simulink model "app_Main100msMgr"  (R2016b)
settings: Solver=FixedStepDiscrete  StartTime=0.0  StopTime=10.0  FixedStep=0.001  RelTol=1e-3  EnableMultiTasking=on
PreLoadFcn:
  | try
  |    tapas_types('load');
  | catch
  |   disp('TAPAS WARNING: Tapas Types could not be loaded ...');
  | end
  | 
  | try
  |   app_types('load');
  | catch
  |   currdir =pwd;
  |   try
  |     cd('..\app_types\');
  |     app_types('load');
  |     cd(currdir);
  |   catch
  |     try
  |        cd('..\..\app_types\');
  |        app_types('load');
  |        cd(currdir);
  |     catch
  |        cd(currdir);
  |        disp('TAPAS WARNING: Application Types could not be loaded ...');
  |     end
  |   end
  |   try
  |       clear currdir;
  |   catch
  |      %Do nothing
  |   end
  | end
libraries: Lib_ICAT_VCU_Com x76, Lib_ICAT_VCU_IO x12, simulink x2, Lib_ICAT_VCU_Anlg x1
(part 1 of 2)
settings Model: Creator=kmansour  LastModifiedBy=Santosh
settings DataIOCC: LimitDataPoints=on  SaveFormat=Array
settings OptimizationCC: LifeSpan=1
settings DebuggingCC: AllowSymbolicDim=off  SFUnexpectedBacktrackingDiag=warning  SFNoUnconditionalDefaultTransitionDiag=warning  SFExecutionAtInitializationDiag=none
settings HardwareCC: ProdBitPerPointer=32  ProdBitPerSizeT=32  ProdBitPerPtrDiffT=32  ProdLargestAtomicInteger=Long  ProdLargestAtomicFloat=Double  ProdWordSize=32  ProdHWDeviceType=Texas Instruments->TMS570 Cortex-R4
settings ModelReferenceCC: ModelReferenceNumInstancesAllowed=Single  PropagateSignalLabelsOutOfModel=off
settings RTWCC: SystemTargetFile=ert.tlc  GenCodeOnly=on  TemplateMakefile=ert_default_tmf  Description=Embedded Coder  GenerateReport=on  IncludeHyperlinkInReport=on  LaunchReport=on  GenerateTraceInfo=on  GenerateTraceReport=on  GenerateTraceReportSl=on  GenerateTraceReportSf=on  GenerateTraceReportEml=on
settings CodeAppCC: IgnoreCustomStorageClasses=off  MaxIdLength=63
settings ERTTargetCC: GenerateSampleERTMain=on  ERTSrcFileBannerTemplate=tapas_code_template.cgt  ERTHdrFileBannerTemplate=tapas_code_template.cgt  ERTDataSrcFileTemplate=tapas_code_template.cgt  ERTDataHdrFileTemplate=tapas_code_template.cgt  ERTCustomFileTemplate=example_file_process.tlc  ConvertIfToSwitch=off  SuppressUnreachableDefaultCases=off
settings ConfigComp: CovMetricSettings=dw  CovHtmlReporting=on  CovSaveCumulativeToWorkspaceVar=on  CovSaveSingleToWorkspaceVar=on  CovExternalEMLEnable=off

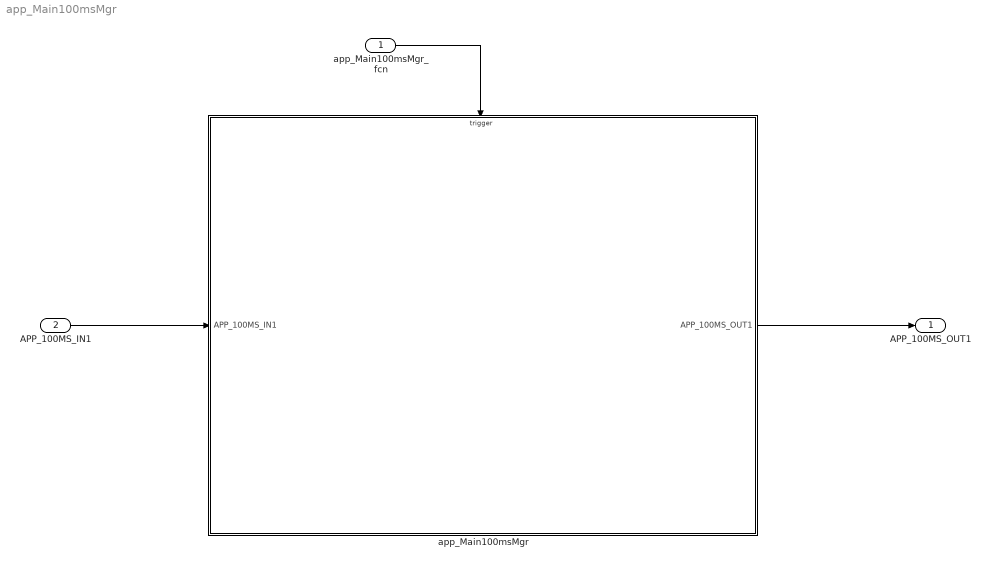
== system app_Main100msMgr ==
  app_Main100msMgr_fcn : Inport  SampleTime=100e-3  OutputFunctionCall=on
  APP_100MS_IN1 : Inport  Port=2
  app_Main100msMgr : Subsystem
  APP_100MS_OUT1 : Outport
  wires:
  app_Main100msMgr_fcn/1 -> app_Main100msMgr/Trigger
  APP_100MS_IN1/1 -> app_Main100msMgr/1(APP_100MS_IN1)
  app_Main100msMgr/1(APP_100MS_OUT1) -> APP_100MS_OUT1/1

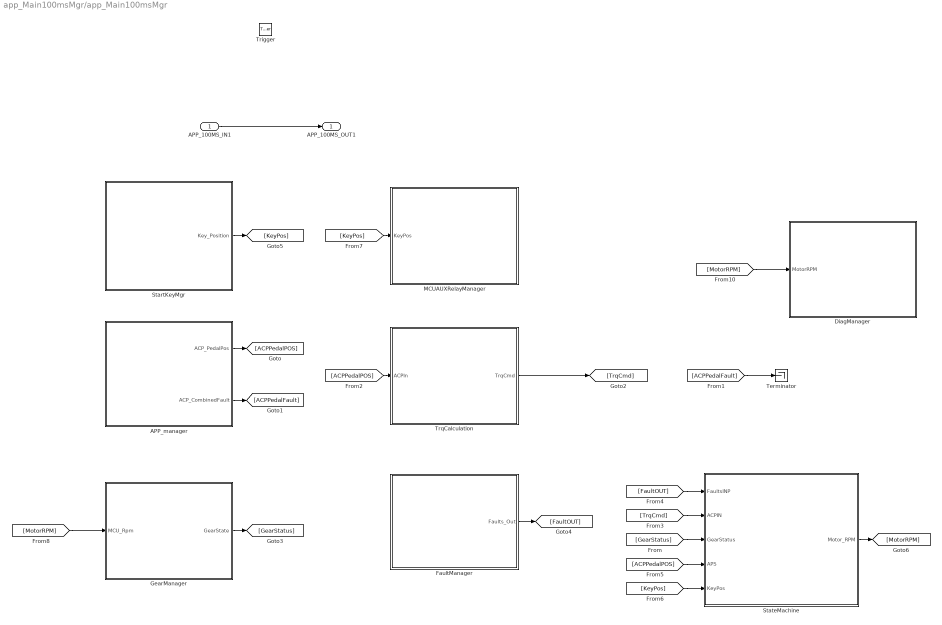
== system app_Main100msMgr/app_Main100msMgr ==
  APP_100MS_IN1 : Inport
  Trigger : TriggerPort  TriggerType=function-call  VariantControl=Variant  SampleTimeType=periodic  SampleTime=-1  PortDimensions=1
  APP_manager : Subsystem
  DiagManager : Subsystem
  FaultManager : Subsystem
  GearManager : Subsystem
  MCUAUXRelayManager : Subsystem
  StartKeyMgr : Subsystem
  StateMachine : Subsystem
  Terminator : Terminator
  TrqCalculation : Subsystem
  APP_100MS_OUT1 : Outport
  wires:
  APP_100MS_IN1/1 -> APP_100MS_OUT1/1
  [ACPPedalPOS] -> StateMachine/4(APS)
  [TrqCmd] -> StateMachine/2(ACPIN)
  [FaultOUT] -> StateMachine/1(FaultsINP)
  [ACPPedalPOS] -> TrqCalculation/1(ACPIn)
  [ACPPedalFault] -> Terminator/1
  GearManager/1(GearState) -> [GearStatus]
  StartKeyMgr/1(Key_Position) -> [KeyPos]
  [KeyPos] -> MCUAUXRelayManager/1(KeyPos)
  [GearStatus] -> StateMachine/3(GearStatus)
  APP_manager/2(ACP_CombinedFault) -> [ACPPedalFault]
  [MotorRPM] -> GearManager/1(MCU_Rpm)
  [MotorRPM] -> DiagManager/1(MotorRPM)
  APP_manager/1(ACP_PedalPos) -> [ACPPedalPOS]
  TrqCalculation/1(TrqCmd) -> [TrqCmd]
  StateMachine/1(Motor_RPM) -> [MotorRPM]
  FaultManager/1(Faults_Out) -> [FaultOUT]
  [KeyPos] -> StateMachine/5(KeyPos)

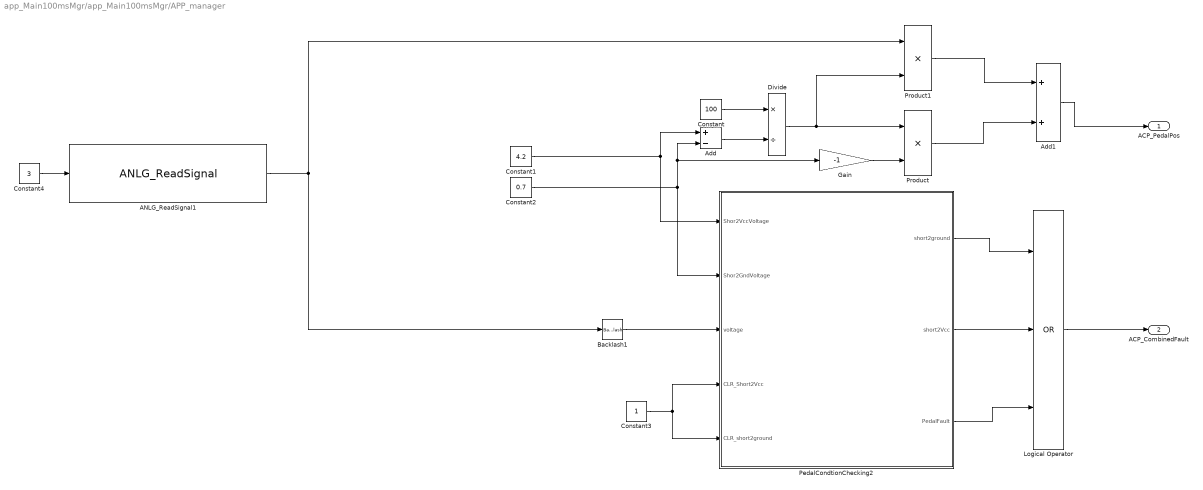
== system app_Main100msMgr/app_Main100msMgr/APP_manager ==
  ANLG_ReadSignal1 : Lib_ICAT_VCU_Anlg/ANLG_ReadSignal  PARAM_ID=ECU_GAS1_ADC_P67
  Add : Sum  Inputs=+-
  Add1 : Sum
  Backlash1 : Backlash  BacklashWidth=5
  Constant : Constant  Value=100
  Constant1 : Constant  Value=4.2
  Constant2 : Constant  Value=0.7
  Constant3 : Constant
  Constant4 : Constant  Value=3
  Divide : Product  Inputs=*/
  Gain : Gain  Gain=-1
  Logical Operator : Logic  Operator=OR  Inputs=3  AllPortsSameDT=off  OutDataTypeStr=boolean
  PedalCondtionChecking2 : Stateflow chart  TreatAsAtomicUnit=on
  Product : Product
  Product1 : Product
  ACP_PedalPos : Outport
  ACP_CombinedFault : Outport  Port=2
  wires:
  PedalCondtionChecking2/3(PedalFault) -> Logical Operator/3
  Constant/1 -> Divide/1
  Constant2/1 -> PedalCondtionChecking2/2(Shor2GndVoltage), Gain/1, Add/2
  ANLG_ReadSignal1/1 -> Backlash1/1, Product1/1
  PedalCondtionChecking2/2(short2Vcc) -> Logical Operator/2
  Backlash1/1 -> PedalCondtionChecking2/3(voltage)
  Logical Operator/1 -> ACP_CombinedFault/1
  Product1/1 -> Add1/1
  Product/1 -> Add1/2
  Divide/1 -> Product1/2, Product/1
  Constant1/1 -> PedalCondtionChecking2/1(Shor2VccVoltage), Add/1
  Gain/1 -> Product/2
  Constant3/1 -> PedalCondtionChecking2/5(CLR_short2ground), PedalCondtionChecking2/4(CLR_Short2Vcc)
  Add/1 -> Divide/2
  Add1/1 -> ACP_PedalPos/1
  PedalCondtionChecking2/1(short2ground) -> Logical Operator/1
  Constant4/1 -> ANLG_ReadSignal1/1

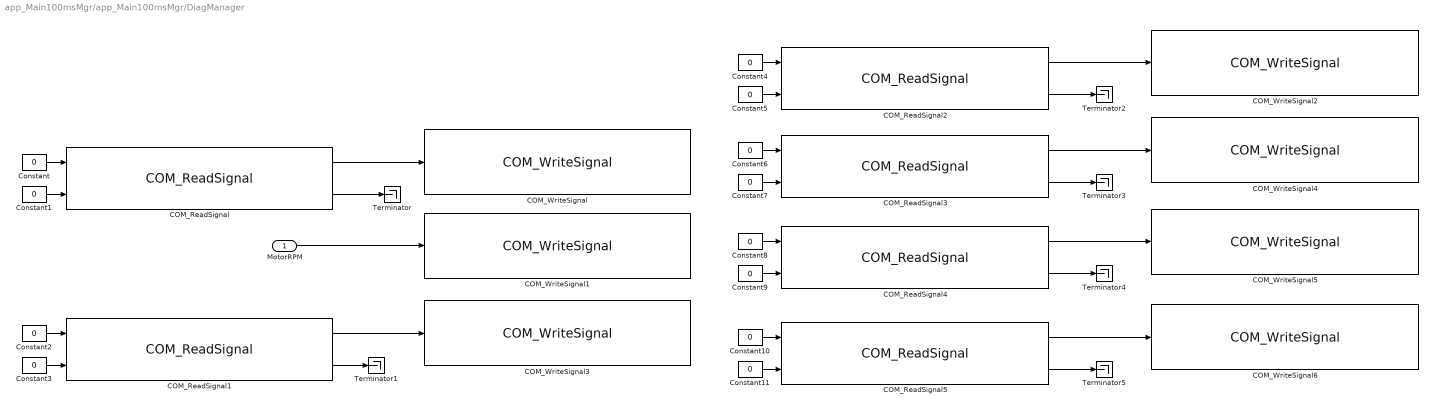
== system app_Main100msMgr/app_Main100msMgr/DiagManager ==
  MotorRPM : Inport
  COM_ReadSignal : Lib_ICAT_VCU_Com/COM_ReadSignal  PARAM_ID=APP_RX_MCU_VCU_ERRORSTATUS_RX1_11
  COM_ReadSignal1 : Lib_ICAT_VCU_Com/COM_ReadSignal  PARAM_ID=APP_RX_MCU_VCU_MOTORTEMP_RX1_3
  COM_ReadSignal2 : Lib_ICAT_VCU_Com/COM_ReadSignal  PARAM_ID=APP_RX_BATTERY_AVER_TEMPER_RX6_2
  COM_ReadSignal3 : Lib_ICAT_VCU_Com/COM_ReadSignal  PARAM_ID=APP_RX_BATTERY_CURRENT_RX6_4
  COM_ReadSignal4 : Lib_ICAT_VCU_Com/COM_ReadSignal  PARAM_ID=APP_RX_BATTERY_VOLTAGE_RX6_5
  COM_ReadSignal5 : Lib_ICAT_VCU_Com/COM_ReadSignal  PARAM_ID=APP_RX_SOC_RX6_3
  COM_WriteSignal : Lib_ICAT_VCU_Com/COM_WriteSignal  PARAM_ID=APP_TX_VCU_HMI_MCUERRORSTATUS_TX8_2
  COM_WriteSignal1 : Lib_ICAT_VCU_Com/COM_WriteSignal  PARAM_ID=APP_TX_VCU_HMI_MOTORRPM_TX8_4
  COM_WriteSignal2 : Lib_ICAT_VCU_Com/COM_WriteSignal  PARAM_ID=APP_TX_VCU_HMI_BATTERY_AVER_TEMP_TX9_4
  COM_WriteSignal3 : Lib_ICAT_VCU_Com/COM_WriteSignal  PARAM_ID=APP_TX_VCU_HMI_MOTORTEMP_TX8_3
  COM_WriteSignal4 : Lib_ICAT_VCU_Com/COM_WriteSignal  PARAM_ID=APP_TX_VCU_HMI_BATTERY_CURRENT_TX9_3
  COM_WriteSignal5 : Lib_ICAT_VCU_Com/COM_WriteSignal  PARAM_ID=APP_TX_VCU_HMI_BATTERY_VOLTAGE_TX9_2
  COM_WriteSignal6 : Lib_ICAT_VCU_Com/COM_WriteSignal  PARAM_ID=APP_TX_VCU_HMI_SOC_TX9_1
  Constant{,1..11} (12 alike) : Constant  Value=0
  Terminator{,1..5} (6 alike) : Terminator
  wires:
  COM_ReadSignal/1 -> COM_WriteSignal/1
  Constant/1 -> COM_ReadSignal/1
  Constant1/1 -> COM_ReadSignal/2
  COM_ReadSignal/2 -> Terminator/1
  MotorRPM/1 -> COM_WriteSignal1/1
  COM_ReadSignal1/1 -> COM_WriteSignal3/1
  COM_ReadSignal1/2 -> Terminator1/1
  Constant3/1 -> COM_ReadSignal1/2
  Constant2/1 -> COM_ReadSignal1/1
  COM_ReadSignal2/2 -> Terminator2/1
  Constant5/1 -> COM_ReadSignal2/2
  Constant4/1 -> COM_ReadSignal2/1
  COM_ReadSignal2/1 -> COM_WriteSignal2/1
  COM_ReadSignal3/1 -> COM_WriteSignal4/1
  Constant6/1 -> COM_ReadSignal3/1
  Constant7/1 -> COM_ReadSignal3/2
  COM_ReadSignal3/2 -> Terminator3/1
  COM_ReadSignal4/2 -> Terminator4/1
  Constant9/1 -> COM_ReadSignal4/2
  Constant8/1 -> COM_ReadSignal4/1
  COM_ReadSignal4/1 -> COM_WriteSignal5/1
  COM_ReadSignal5/1 -> COM_WriteSignal6/1
  Constant10/1 -> COM_ReadSignal5/1
  Constant11/1 -> COM_ReadSignal5/2
  COM_ReadSignal5/2 -> Terminator5/1

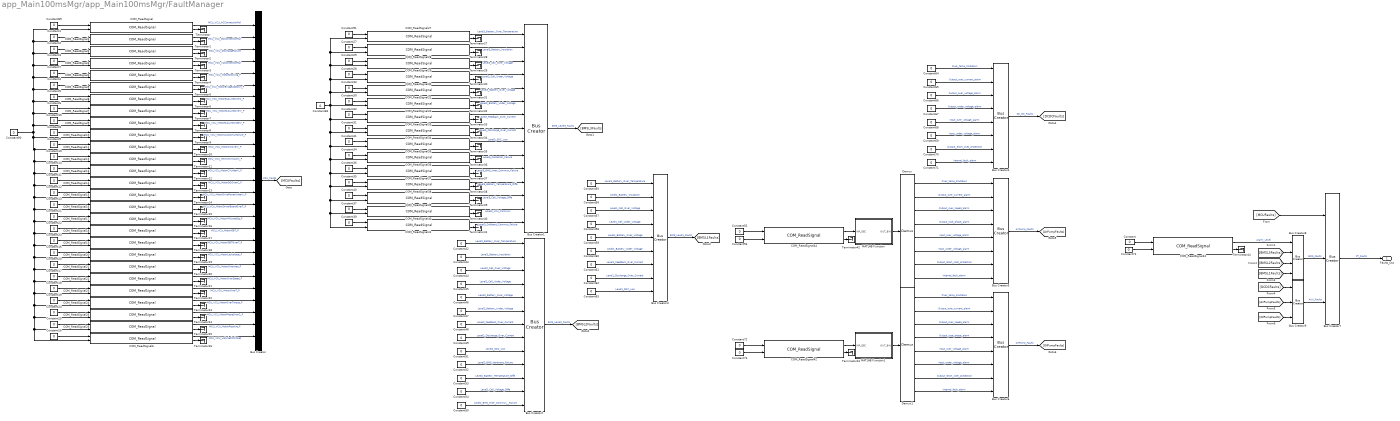
== system app_Main100msMgr/app_Main100msMgr/FaultManager ==
  Bus Creator : BusCreator  Inputs=27
  Bus Creator1 : BusCreator  Inputs=15
  Bus Creator2 : BusCreator  Inputs=13
  Bus Creator3 : BusCreator  Inputs=9
  Bus Creator4 : BusCreator  Inputs=8
  Bus Creator5 : BusCreator  Inputs=8
  Bus Creator6 : BusCreator  Inputs=8
  Bus Creator7 : BusCreator  Inputs=3
  Bus Creator8 : BusCreator  Inputs=4
  Bus Creator9 : BusCreator  Inputs=3
  COM_ReadSignal : Lib_ICAT_VCU_Com/COM_ReadSignal  PARAM_ID=APP_RX_MCU_VCU_ACCONNECTIONFAIL_RX4_3
  COM_ReadSignal1 : Lib_ICAT_VCU_Com/COM_ReadSignal  PARAM_ID=APP_RX_MCU_VCU_DCCONNECTIONFAIL_RX4_2
  COM_ReadSignal10 : Lib_ICAT_VCU_Com/COM_ReadSignal  PARAM_ID=APP_RX_MCU_VCU_MOTORCANCOMFAIL_P_RX4_6
  COM_ReadSignal11 : Lib_ICAT_VCU_Com/COM_ReadSignal  PARAM_ID=APP_RX_MCU_VCU_MOTORCVOVERV_P_RX4_13
  COM_ReadSignal12 : Lib_ICAT_VCU_Com/COM_ReadSignal  PARAM_ID=APP_RX_MCU_VCU_MTRCVRVRCONN_P_RX4_12
  COM_ReadSignal13 : Lib_ICAT_VCU_Com/COM_ReadSignal  PARAM_ID=APP_RX_MCU_VCU_MOTORCVUNDERV_P_RX4_27
  COM_ReadSignal14 : Lib_ICAT_VCU_Com/COM_ReadSignal  PARAM_ID=APP_RX_MCU_VCU_MOTORDQOVERC_P_RX4_14
  COM_ReadSignal15 : Lib_ICAT_VCU_Com/COM_ReadSignal  PARAM_ID=APP_RX_MCU_VCU_MTRDRVPWRUNDRV_P_RX4_21
  COM_ReadSignal16 : Lib_ICAT_VCU_Com/COM_ReadSignal  PARAM_ID=APP_RX_MCU_VCU_MTRDRVRBRDOVRT_P_RX4_4
  COM_ReadSignal17 : Lib_ICAT_VCU_Com/COM_ReadSignal  PARAM_ID=APP_RX_MCU_VCU_MOTORHWLOSESIG_P_RX4_10
  COM_ReadSignal18 : Lib_ICAT_VCU_Com/COM_ReadSignal  PARAM_ID=APP_RX_MCU_VCU_MOTORIGBT_P_RX4_20
  COM_ReadSignal19 : Lib_ICAT_VCU_Com/COM_ReadSignal  PARAM_ID=APP_RX_MCU_VCU_MOTORIGBTOVERT_P_RX4_23
  COM_ReadSignal2 : Lib_ICAT_VCU_Com/COM_ReadSignal  PARAM_ID=APP_RX_MCU_VCU_DISCHARGEFAILURE_RX4_11
  COM_ReadSignal20 : Lib_ICAT_VCU_Com/COM_ReadSignal  PARAM_ID=APP_RX_MCU_VCU_MOTORLACKPHASE_P_RX4_8
  COM_ReadSignal21 : Lib_ICAT_VCU_Com/COM_ReadSignal  PARAM_ID=APP_RX_MCU_VCU_MOTOROVERLOAD_P_RX4_18
  COM_ReadSignal22 : Lib_ICAT_VCU_Com/COM_ReadSignal  PARAM_ID=APP_RX_MCU_VCU_MOTOROVERSPEED_P_RX4_5
  COM_ReadSignal23 : Lib_ICAT_VCU_Com/COM_ReadSignal  PARAM_ID=APP_RX_MCU_VCU_MOTOROVERT_P_RX4_24
  COM_ReadSignal24 : Lib_ICAT_VCU_Com/COM_ReadSignal  PARAM_ID=APP_RX_MCU_VCU_MOTOROVERTORQUE_P_RX4_17
  COM_ReadSignal25 : Lib_ICAT_VCU_Com/COM_ReadSignal  PARAM_ID=APP_RX_MCU_VCU_MOTORPHASEOVERC_P_RX4_26
  COM_ReadSignal26 : Lib_ICAT_VCU_Com/COM_ReadSignal  PARAM_ID=APP_RX_MCU_VCU_MOTORRESOLVE_P_RX4_9
  COM_ReadSignal27 : Lib_ICAT_VCU_Com/COM_ReadSignal  PARAM_ID=APP_RX_LEVEL3_BATT_OVER_TEMP_RX16_25
  COM_ReadSignal28 : Lib_ICAT_VCU_Com/COM_ReadSignal  PARAM_ID=APP_RX_LEVEL3_BATT_INSULATION_RX16_24
  COM_ReadSignal29 : Lib_ICAT_VCU_Com/COM_ReadSignal  PARAM_ID=APP_RX_LEVEL3_CELL_OVER_VOLTAGE_RX16_30
  COM_ReadSignal3 : Lib_ICAT_VCU_Com/COM_ReadSignal  PARAM_ID=APP_RX_MCU_VCU_K2CONNECTIONFAIL_RX4_1
  COM_ReadSignal30 : Lib_ICAT_VCU_Com/COM_ReadSignal  PARAM_ID=APP_RX_LEVEL3_CELL_UNDER_VTG_RX16_31
  COM_ReadSignal31 : Lib_ICAT_VCU_Com/COM_ReadSignal  PARAM_ID=APP_RX_LEVEL3_BATT_OVER_VTG_RX16_26
  COM_ReadSignal32 : Lib_ICAT_VCU_Com/COM_ReadSignal  PARAM_ID=APP_RX_LEVEL3_BATT_UNDER_VTG_RX16_28
  COM_ReadSignal33 : Lib_ICAT_VCU_Com/COM_ReadSignal  PARAM_ID=APP_RX_LEVEL3_FBKOVERCURR_RX16_35
  COM_ReadSignal34 : Lib_ICAT_VCU_Com/COM_ReadSignal  PARAM_ID=APP_RX_LEVEL3_DIS_OVER_CURR_RX16_34
  COM_ReadSignal35 : Lib_ICAT_VCU_Com/COM_ReadSignal  PARAM_ID=APP_RX_LEVEL3_SOC_LOW_RX16_37
  COM_ReadSignal36 : Lib_ICAT_VCU_Com/COM_ReadSignal  PARAM_ID=APP_RX_LEVEL3_CONTACTOR_FAILURE_RX16_33
  COM_ReadSignal37 : Lib_ICAT_VCU_Com/COM_ReadSignal  PARAM_ID=APP_RX_LEVEL3_BMSINNERCOMMFAIL_RX16_29
  COM_ReadSignal38 : Lib_ICAT_VCU_Com/COM_ReadSignal  PARAM_ID=APP_RX_LEVEL3_BATT_TEMP_DIFFE_RX16_27
  COM_ReadSignal39 : Lib_ICAT_VCU_Com/COM_ReadSignal  PARAM_ID=APP_RX_LEVEL3_CELL_VTG_DIFFE_RX16_32
  COM_ReadSignal4 : Lib_ICAT_VCU_Com/COM_ReadSignal  PARAM_ID=APP_RX_MCU_VCU_MOTORBLOCKING_P_RX4_19
  COM_ReadSignal40 : Lib_ICAT_VCU_Com/COM_ReadSignal  PARAM_ID=APP_RX_LEVEL3_VCU_COMMUN_RX16_38
  COM_ReadSignal41 : Lib_ICAT_VCU_Com/COM_ReadSignal  PARAM_ID=APP_RX_LEVEL3_ONBOARDCOMMFAIL_RX16_36
  COM_ReadSignal42 : Lib_ICAT_VCU_Com/COM_ReadSignal  PARAM_ID=APP_RX_AUX_VCU_OILPUMP_FAULT_RX20_1
  COM_ReadSignal43 : Lib_ICAT_VCU_Com/COM_ReadSignal  PARAM_ID=APP_RX_AUX_VCU_OILPUMP_FAULT_RX20_1
  COM_ReadSignal44 : Lib_ICAT_VCU_Com/COM_ReadSignal  PARAM_ID=APP_RX_AUX_VCU_AIRPUMP_FAULT_RX19_1
  COM_ReadSignal5 : Lib_ICAT_VCU_Com/COM_ReadSignal  PARAM_ID=APP_RX_MCU_VCU_MOTORBRDGUPDWN_P_RX4_22
  COM_ReadSignal6 : Lib_ICAT_VCU_Com/COM_ReadSignal  PARAM_ID=APP_RX_MCU_VCU_VEHICLEFAULTCKTRES_RX4_7
  COM_ReadSignal7 : Lib_ICAT_VCU_Com/COM_ReadSignal  PARAM_ID=APP_RX_MCU_VCU_MTRBUSLINEOVERV_P_RX4_16
  COM_ReadSignal8 : Lib_ICAT_VCU_Com/COM_ReadSignal  PARAM_ID=APP_RX_MCU_VCU_MTRBUSLINEOVRC_P_RX4_25
  COM_ReadSignal9 : Lib_ICAT_VCU_Com/COM_ReadSignal  PARAM_ID=APP_RX_MCU_VCU_MTRBUSLINEUNDRV_P_RX4_15
  Constant{,1..74,89..93} (80 alike) : Constant  Value=0
  Demux : Demux  Outputs=8
  Demux1 : Demux  Outputs=8
  MATLAB Function : MATLAB Function  TreatAsAtomicUnit=on
  MATLAB Function1 : MATLAB Function  TreatAsAtomicUnit=on
  Terminator{,1..44} (45 alike) : Terminator
  Faults_Out : Outport
  wires:
  COM_ReadSignal/1 -> Bus Creator/1  "MCU_VCU_ACConnectionFail"
  COM_ReadSignal1/1 -> Bus Creator/2  "MCU_VCU_DCConnectionFail"
  COM_ReadSignal2/1 -> Bus Creator/3  "MCU_VCU_DischargeFailure"
  COM_ReadSignal3/1 -> Bus Creator/4  "MCU_VCU_K2ConnectionFail"
  COM_ReadSignal8/1 -> Bus Creator/7  "MCU_VCU_MotorBusLineOverC_P"
  COM_ReadSignal7/1 -> Bus Creator/8  "MCU_VCU_MotorBusLineOverV_P"
  COM_ReadSignal5/1 -> Bus Creator/6  "MCU_VCU_MotorBridgeUpDown_P"
  COM_ReadSignal4/1 -> Bus Creator/5  "MCU_VCU_MotorBlocking_P"
  COM_ReadSignal11/1 -> Bus Creator/11  "MCU_VCU_MotorCVOverV_P"
  COM_ReadSignal9/1 -> Bus Creator/9  "MCU_VCU_MotorBusLineUnderV_P"
  COM_ReadSignal10/1 -> Bus Creator/10  "MCU_VCU_MotorCANComuiFailure_P"
  COM_ReadSignal12/1 -> Bus Creator/12  "MCU_VCU_MtrCVRvrsConn_P"
  COM_ReadSignal13/1 -> Bus Creator/13  "MCU_VCU_MotorCVUnderV_P"
  COM_ReadSignal14/1 -> Bus Creator/14  "MCU_VCU_MotorDQOverC_P"
  COM_ReadSignal15/1 -> Bus Creator/15  "MCU_VCU_MotorDrivePowerUnderV_P"
  COM_ReadSignal16/1 -> Bus Creator/16  "MCU_VCU_MotorDriverBoardOverT_P"
  COM_ReadSignal26/1 -> Bus Creator/26  "MCU_VCU_MotorResolve_P"
  COM_ReadSignal25/1 -> Bus Creator/25  "MCU_VCU_MotorPhaseOverC_P"
  COM_ReadSignal24/1 -> Bus Creator/24  "MCU_VCU_MotorOverTorque_P"
  COM_ReadSignal23/1 -> Bus Creator/23  "MCU_VCU_MotorOverT_P"
  COM_ReadSignal22/1 -> Bus Creator/22  "MCU_VCU_MotorOverSpeed_P"
  COM_ReadSignal20/1 -> Bus Creator/20  "MCU_VCU_MotorLackphase_P"
  COM_ReadSignal19/1 -> Bus Creator/19  "MCU_VCU_MotorIGBTOverT_P"
  COM_ReadSignal21/1 -> Bus Creator/21  "MCU_VCU_MotorOverload_P"
  COM_ReadSignal18/1 -> Bus Creator/18  "MCU_VCU_MotorIGBT_P"
  COM_ReadSignal17/1 -> Bus Creator/17  "MCU_VCU_MotorHWLoseSig_P"
  COM_ReadSignal6/1 -> Bus Creator/27  "MCU_VCU_VehicleFltCktRes"
  COM_ReadSignal27/1 -> Bus Creator1/1  "Level3_Battery_Over_Temperature"
  COM_ReadSignal28/1 -> Bus Creator1/2  "Level3_Battery_Insulation"
  COM_ReadSignal29/1 -> Bus Creator1/3  "Level3_Cell_Over_Voltage"
  COM_ReadSignal30/1 -> Bus Creator1/4  "Level3_Cell_Under_Voltage"
  COM_ReadSignal31/1 -> Bus Creator1/5  "Level3_Battery_Over_Voltage"
  COM_ReadSignal32/1 -> Bus Creator1/6  "Level3_Battery_Under_Voltage"
  COM_ReadSignal33/1 -> Bus Creator1/7  "Level3_Feedback_Over_Current"
  COM_ReadSignal34/1 -> Bus Creator1/8  "Level3_Discharge_Over_Current"
  COM_ReadSignal35/1 -> Bus Creator1/9  "Level3_SOC_Low"
  COM_ReadSignal40/1 -> Bus Creator1/14  "Level3_VCU_Commun"
  COM_ReadSignal39/1 -> Bus Creator1/13  "Level3_Cell_Voltage_Diffe"
  COM_ReadSignal38/1 -> Bus Creator1/12  "Level3_Battery_Temperature_Diffe"
  COM_ReadSignal37/1 -> Bus Creator1/11  "Level3_BMS_Inner_Commun_Failure"
  COM_ReadSignal36/1 -> Bus Creator1/10  "Level3_Contactor_Failure"
  COM_ReadSignal41/1 -> Bus Creator1/15  "Level3_OnBoard_Commun_Failure"
  Constant51/1 -> Bus Creator2/9  "Level2_SOC_Low"
  Constant52/1 -> Bus Creator2/10  "Level2_BMS_Hardware_Failure"
  Constant53/1 -> Bus Creator2/11  "Level2_Battery_Temperature_Diffe"
  Constant54/1 -> Bus Creator2/12  "Level2_Cell_Voltage_Diffe"
  Constant50/1 -> Bus Creator2/13  "Level2_BMS_Inner_Commun__Failure"
  Constant49/1 -> Bus Creator2/8  "Level2_Discharge_Over_Current"
  Constant48/1 -> Bus Creator2/7  "Level2_Feedback_Over_Current"
  Constant47/1 -> Bus Creator2/6  "Level2_Battery_Under_Voltage"
  Constant46/1 -> Bus Creator2/5  "Level2_Battery_Over_Voltage"
  Constant45/1 -> Bus Creator2/4  "Level2_Cell_Under_Voltage"
  Constant44/1 -> Bus Creator2/3  "Level2_Cell_Over_Voltage"
  Constant43/1 -> Bus Creator2/2  "Level2_Battery_Insulation"
  Constant42/1 -> Bus Creator2/1  "Level2_Battery_Over_Temperature"
  Constant55/1 -> Bus Creator3/1  "Level1_Battery_Over_Temperature"
  Constant56/1 -> Bus Creator3/2  "Level1_Battery_Insulation"
  Constant57/1 -> Bus Creator3/3  "Level1_Cell_Over_Voltage"
  Constant58/1 -> Bus Creator3/4  "Level1_Cell_Under_Voltage"
  Constant59/1 -> Bus Creator3/5  "Level1_Battery_Over_Voltage"
  Constant60/1 -> Bus Creator3/6  "Level1_Battery_Under_Voltage"
  Constant61/1 -> Bus Creator3/7  "Level1_Feedback_Over_Current"
  Constant62/1 -> Bus Creator3/8  "Level1_Discharge_Over_Current"
  Constant63/1 -> Bus Creator3/9  "Level1_SOC_Low"
  Bus Creator/1 -> [MCUFaults]  "MCU_Faults"
  Bus Creator1/1 -> [BMSL3Faults]  "BMS_Level3_Faults"
  Bus Creator2/1 -> [BMSL2Faults]  "BMS_Level2_Faults"
  Bus Creator3/1 -> [BMSL1Faults]  "BMS_Level1_Faults"
  Constant71/1 -> Bus Creator4/8  "internal_fault_alarm"
  Constant70/1 -> Bus Creator4/7  "Output_Short_cket_protection"
  Constant69/1 -> Bus Creator4/6  "Input_under_voltage_alarm"
  Constant68/1 -> Bus Creator4/5  "Input_over_voltage_alarm"
  Constant67/1 -> Bus Creator4/4  "Output_under_voltage_alarm"
  Constant66/1 -> Bus Creator4/3  "Output_over_voltage_alarm"
  Constant65/1 -> Bus Creator4/2  "Output_over_current_alarm"
  Constant64/1 -> Bus Creator4/1  "Over_temp_shutdown"
  Bus Creator4/1 -> [DCDCFaults]  "DC_DC_Faults"
  Bus Creator5/1 -> [AirPumpFaults]  "AirPump_Faults"
  Demux/1 -> Bus Creator5/1  "Over_temp_shutdown"
  Demux/2 -> Bus Creator5/2  "Output_over_current_alarm"
  Demux/3 -> Bus Creator5/3  "Output_over_speed_alarm"
  Demux/4 -> Bus Creator5/4  "Output_lose_phase_alarm"
  Demux/5 -> Bus Creator5/5  "Input_over_voltage_alarm"
  Demux/6 -> Bus Creator5/6  "Input_under_voltage_alarm"
  Demux/7 -> Bus Creator5/7  "Output_Short_cket_protection"
  Demux/8 -> Bus Creator5/8  "internal_fault_alarm"
  Demux1/8 -> Bus Creator6/8  "internal_fault_alarm"
  Demux1/7 -> Bus Creator6/7  "Output_Short_cket_protection"
  Demux1/6 -> Bus Creator6/6  "Input_under_voltage_alarm"
  Demux1/5 -> Bus Creator6/5  "Input_over_voltage_alarm"
  Demux1/4 -> Bus Creator6/4  "Output_lose_phase_alarm"
  Demux1/3 -> Bus Creator6/3  "Output_over_speed_alarm"
  Demux1/2 -> Bus Creator6/2  "Output_over_current_alarm"
  Demux1/1 -> Bus Creator6/1  "Over_temp_shutdown"
  Bus Creator6/1 -> [OilPumpFaults]  "OilPump_Faults"
  [MCUFaults] -> Bus Creator7/1
  Bus Creator7/1 -> Faults_Out/1  "PT_Faults"
  [OilPumpFaults] -> Bus Creator9/3
  [AirPumpFaults] -> Bus Creator9/2
  [DCDCFaults] -> Bus Creator9/1
  Bus Creator8/1 -> Bus Creator7/2  "BMS_Faults"
  Bus Creator9/1 -> Bus Creator7/3  "AUX_Faults"
  [BMSL1Faults] -> Bus Creator8/4
  [BMSL2Faults] -> Bus Creator8/3
  [BMSL3Faults] -> Bus Creator8/2
  COM_ReadSignal43/1 -> Bus Creator8/1  "Alarm_Level"
  Constant89/1 -> COM_ReadSignal/1
  COM_ReadSignal/2 -> Terminator/1
  COM_ReadSignal1/2 -> Terminator1/1
  Constant1/1 -> COM_ReadSignal1/1
  COM_ReadSignal2/2 -> Terminator2/1
  COM_ReadSignal3/2 -> Terminator3/1
  COM_ReadSignal4/2 -> Terminator4/1
  COM_ReadSignal5/2 -> Terminator5/1
  COM_ReadSignal8/2 -> Terminator6/1
  COM_ReadSignal7/2 -> Terminator7/1
  COM_ReadSignal9/2 -> Terminator8/1
  COM_ReadSignal10/2 -> Terminator9/1
  COM_ReadSignal11/2 -> Terminator10/1
  COM_ReadSignal12/2 -> Terminator11/1
  COM_ReadSignal13/2 -> Terminator12/1
  COM_ReadSignal14/2 -> Terminator13/1
  COM_ReadSignal15/2 -> Terminator14/1
  COM_ReadSignal16/2 -> Terminator15/1
  COM_ReadSignal17/2 -> Terminator16/1
  COM_ReadSignal18/2 -> Terminator17/1
  COM_ReadSignal19/2 -> Terminator18/1
  COM_ReadSignal20/2 -> Terminator19/1
  COM_ReadSignal21/2 -> Terminator20/1
  COM_ReadSignal22/2 -> Terminator21/1
  COM_ReadSignal23/2 -> Terminator22/1
  COM_ReadSignal24/2 -> Terminator23/1
  COM_ReadSignal25/2 -> Terminator24/1
  COM_ReadSignal26/2 -> Terminator25/1
  COM_ReadSignal6/2 -> Terminator26/1
  Constant2/1 -> COM_ReadSignal2/1
  Constant3/1 -> COM_ReadSignal3/1
  Constant7/1 -> COM_ReadSignal4/1
  Constant4/1 -> COM_ReadSignal5/1
  Constant5/1 -> COM_ReadSignal8/1
  Constant6/1 -> COM_ReadSignal7/1
  Constant15/1 -> COM_ReadSignal9/1
  Constant8/1 -> COM_ReadSignal10/1
  Constant9/1 -> COM_ReadSignal11/1
  Constant10/1 -> COM_ReadSignal12/1
  Constant14/1 -> COM_ReadSignal13/1
  Constant11/1 -> COM_ReadSignal14/1
  Constant12/1 -> COM_ReadSignal15/1
  Constant13/1 -> COM_ReadSignal16/1
  Constant21/1 -> COM_ReadSignal17/1
  Constant22/1 -> COM_ReadSignal18/1
  Constant23/1 -> COM_ReadSignal19/1
  Constant16/1 -> COM_ReadSignal20/1
  Constant20/1 -> COM_ReadSignal21/1
  Constant17/1 -> COM_ReadSignal22/1
  Constant18/1 -> COM_ReadSignal23/1
  Constant19/1 -> COM_ReadSignal24/1
  Constant24/1 -> COM_ReadSignal25/1
  Constant25/1 -> COM_ReadSignal26/1
  Constant26/1 -> COM_ReadSignal6/1
  Constant90/1 -> COM_ReadSignal15/2, COM_ReadSignal16/2, COM_ReadSignal17/2, COM_ReadSignal18/2, COM_ReadSignal19/2, COM_ReadSignal20/2, COM_ReadSignal21/2, COM_ReadSignal22/2, COM_ReadSignal23/2, COM_ReadSignal24/2, COM_ReadSignal25/2, COM_ReadSignal26/2, COM_ReadSignal6/2, COM_ReadSignal14/2, COM_ReadSignal13/2, COM_ReadSignal12/2, COM_ReadSignal11/2, COM_ReadSignal10/2, COM_ReadSignal9/2, COM_ReadSignal7/2, COM_ReadSignal8/2, COM_ReadSignal5/2, COM_ReadSignal4/2, COM_ReadSignal3/2, COM_ReadSignal2/2, COM_ReadSignal1/2, COM_ReadSignal/2
  Constant91/1 -> COM_ReadSignal27/1
  COM_ReadSignal27/2 -> Terminator27/1
  Constant27/1 -> COM_ReadSignal28/1
  Constant28/1 -> COM_ReadSignal30/1
  Constant29/1 -> COM_ReadSignal29/1
  Constant32/1 -> COM_ReadSignal33/1
  Constant30/1 -> COM_ReadSignal32/1
  Constant33/1 -> COM_ReadSignal31/1
  Constant31/1 -> COM_ReadSignal34/1
  Constant41/1 -> COM_ReadSignal35/1
  Constant34/1 -> COM_ReadSignal36/1
  Constant36/1 -> COM_ReadSignal37/1
  Constant35/1 -> COM_ReadSignal38/1
  Constant40/1 -> COM_ReadSignal39/1
  Constant37/1 -> COM_ReadSignal40/1
  Constant39/1 -> COM_ReadSignal41/1
  COM_ReadSignal28/2 -> Terminator28/1
  COM_ReadSignal29/2 -> Terminator29/1
  COM_ReadSignal30/2 -> Terminator30/1
  COM_ReadSignal31/2 -> Terminator31/1
  COM_ReadSignal32/2 -> Terminator32/1
  COM_ReadSignal33/2 -> Terminator33/1
  COM_ReadSignal34/2 -> Terminator34/1
  COM_ReadSignal35/2 -> Terminator35/1
  COM_ReadSignal36/2 -> Terminator36/1
  COM_ReadSignal37/2 -> Terminator37/1
  COM_ReadSignal38/2 -> Terminator38/1
  COM_ReadSignal39/2 -> Terminator39/1
  COM_ReadSignal40/2 -> Terminator40/1
  COM_ReadSignal41/2 -> Terminator41/1
  Constant38/1 -> COM_ReadSignal33/2, COM_ReadSignal34/2, COM_ReadSignal35/2, COM_ReadSignal36/2, COM_ReadSignal37/2, COM_ReadSignal38/2, COM_ReadSignal39/2, COM_ReadSignal40/2, COM_ReadSignal41/2, COM_ReadSignal31/2, COM_ReadSignal30/2, COM_ReadSignal29/2, COM_ReadSignal28/2, COM_ReadSignal27/2, COM_ReadSignal32/2
  Constant92/1 -> COM_ReadSignal44/1
  Constant93/1 -> COM_ReadSignal44/2
  MATLAB Function/1(OUT_BIN) -> Demux/1
  COM_ReadSignal44/1 -> MATLAB Function/1(INP_DEC)
  COM_ReadSignal44/2 -> Terminator42/1
  MATLAB Function1/1(OUT_BIN) -> Demux1/1
  COM_ReadSignal42/2 -> Terminator43/1
  COM_ReadSignal42/1 -> MATLAB Function1/1(INP_DEC)
  Constant73/1 -> COM_ReadSignal42/2
  Constant72/1 -> COM_ReadSignal42/1
  Constant/1 -> COM_ReadSignal43/1
  Constant74/1 -> COM_ReadSignal43/2
  COM_ReadSignal43/2 -> Terminator44/1

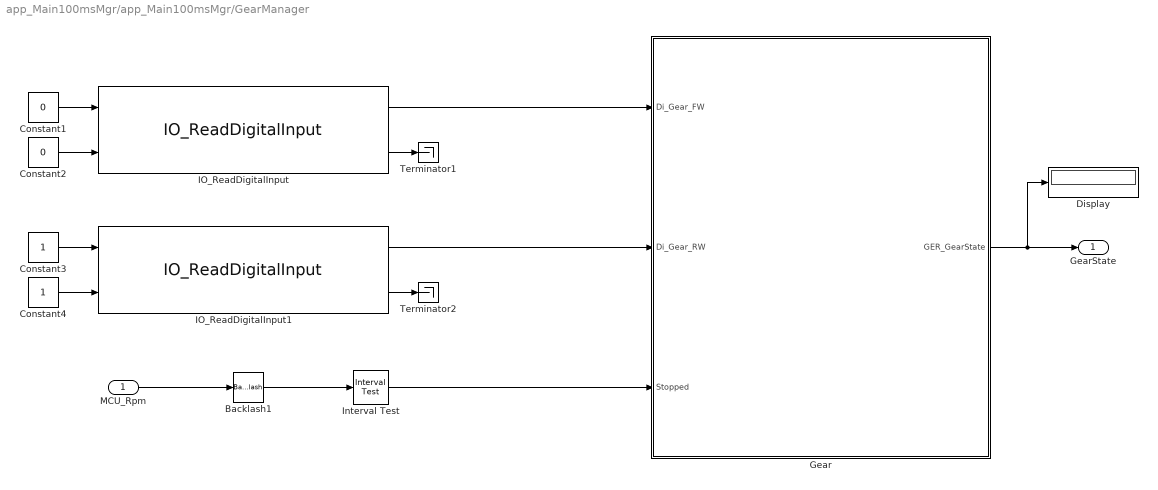
== system app_Main100msMgr/app_Main100msMgr/GearManager ==
  MCU_Rpm : Inport
  Backlash1 : Backlash  BacklashWidth=3
  Constant1 : Constant  Value=0
  Constant2 : Constant  Value=0
  Constant3 : Constant
  Constant4 : Constant
  Display : Display
  Gear : Stateflow chart  TreatAsAtomicUnit=on
  IO_ReadDigitalInput : Lib_ICAT_VCU_IO/IO_ReadDigitalInput  PARAM_ID=ECU_GEAR_D_DI_P25
  IO_ReadDigitalInput1 : Lib_ICAT_VCU_IO/IO_ReadDigitalInput  PARAM_ID=ECU_GEAR_R_DI_P28
  Interval Test : simulink/Logic and Bit Operations/Interval Test  IntervalClosedRight=on  uplimit=4  IntervalClosedLeft=on  lowlimit=-4  OutDataTypeStr=boolean
  Terminator1 : Terminator
  Terminator2 : Terminator
  GearState : Outport
  wires:
  Interval Test/1 -> Gear/3(Stopped)
  IO_ReadDigitalInput/2 -> Terminator1/1
  MCU_Rpm/1 -> Backlash1/1
  IO_ReadDigitalInput/1 -> Gear/1(Di_Gear_FW)
  Backlash1/1 -> Interval Test/1
  Gear/1(GER_GearState) -> Display/1, GearState/1
  Constant1/1 -> IO_ReadDigitalInput/1
  Constant2/1 -> IO_ReadDigitalInput/2
  IO_ReadDigitalInput1/1 -> Gear/2(Di_Gear_RW)
  IO_ReadDigitalInput1/2 -> Terminator2/1
  Constant4/1 -> IO_ReadDigitalInput1/2
  Constant3/1 -> IO_ReadDigitalInput1/1

== system app_Main100msMgr/app_Main100msMgr/MCUAUXRelayManager ==
  KeyPos : Inport
  PDU_4in1_Handler : Subsystem
  wires:
  KeyPos/1 -> PDU_4in1_Handler/1(KeyPos)

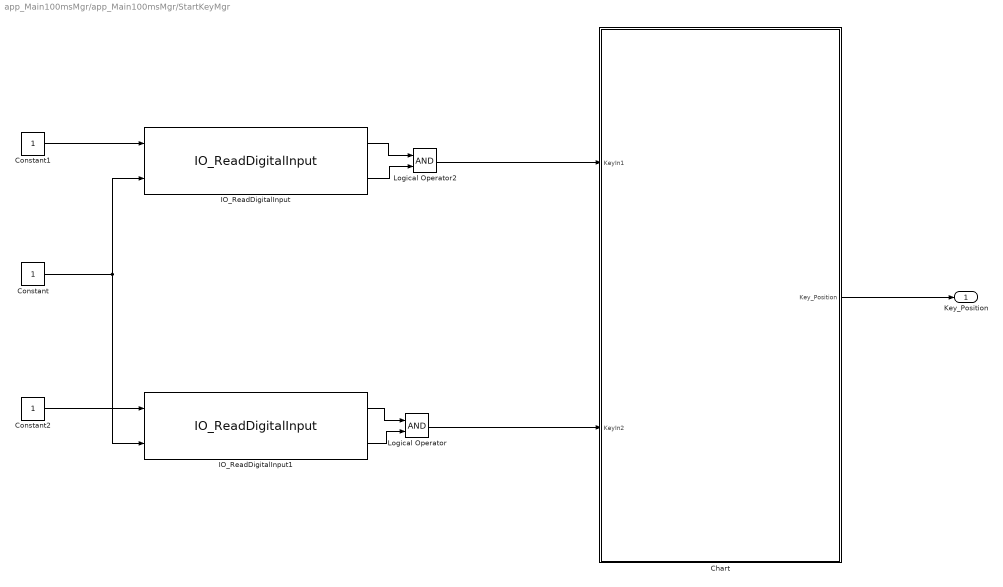
== system app_Main100msMgr/app_Main100msMgr/StartKeyMgr ==
  Chart : Stateflow chart  TreatAsAtomicUnit=on
  Constant : Constant
  Constant1 : Constant
  Constant2 : Constant
  IO_ReadDigitalInput : Lib_ICAT_VCU_IO/IO_ReadDigitalInput  PARAM_ID=ECU_KEY_ACC_DI_P32
  IO_ReadDigitalInput1 : Lib_ICAT_VCU_IO/IO_ReadDigitalInput  PARAM_ID=ECU_KEY_START_DI_P27
  Logical Operator : Logic  AllPortsSameDT=off  OutDataTypeStr=boolean
  Logical Operator2 : Logic  AllPortsSameDT=off  OutDataTypeStr=boolean
  Key_Position : Outport
  wires:
  IO_ReadDigitalInput1/1 -> Logical Operator/1
  IO_ReadDigitalInput1/2 -> Logical Operator/2
  Logical Operator/1 -> Chart/2(KeyIn2)
  IO_ReadDigitalInput/1 -> Logical Operator2/1
  IO_ReadDigitalInput/2 -> Logical Operator2/2
  Logical Operator2/1 -> Chart/1(KeyIn1)
  Constant/1 -> IO_ReadDigitalInput1/2, IO_ReadDigitalInput/2
  Chart/1(Key_Position) -> Key_Position/1
  Constant1/1 -> IO_ReadDigitalInput/1
  Constant2/1 -> IO_ReadDigitalInput1/1

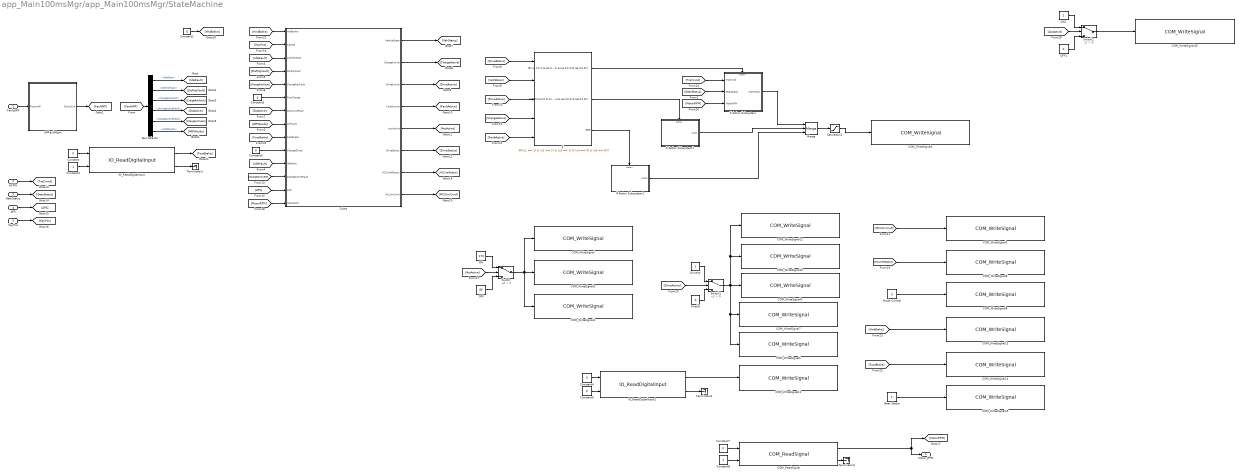
== system app_Main100msMgr/app_Main100msMgr/StateMachine ==
  FaultsINP : Inport
  ACPIN : Inport  Port=2
  GearStatus : Inport  Port=3
  APS : Inport  Port=4
  KeyPos : Inport  Port=5
  Bus Selector : BusSelector  OutputSignals=IdleFault,DisRdyFault,ChargeRdyFault,DrivingActiveFault,ChargeActiveFault,AllPtFaults
  COM_ReadSignal : Lib_ICAT_VCU_Com/COM_ReadSignal  PARAM_ID=APP_RX_MCU_VCU_MOTORRPM_RX1_4
  COM_WriteSignal : Lib_ICAT_VCU_Com/COM_WriteSignal  PARAM_ID=APP_TX_VCU_AUX_AIRPUMP_COMMAND_TX4_1
  COM_WriteSignal1 : Lib_ICAT_VCU_Com/COM_WriteSignal  PARAM_ID=APP_TX_VCU_MCU_TORQUESETPOINT_TX1_8
  COM_WriteSignal10 : Lib_ICAT_VCU_Com/COM_WriteSignal  PARAM_ID=APP_TX_VCU_MCU_K2CLOSEREQUESTVALI_TX1_5
  COM_WriteSignal11 : Lib_ICAT_VCU_Com/COM_WriteSignal  PARAM_ID=APP_TX_VCU_MCU_RELAYK1STATUS_TX1_2
  COM_WriteSignal12 : Lib_ICAT_VCU_Com/COM_WriteSignal  PARAM_ID=APP_TX_VCU_MCU_ESTOPSTATUS_TX1_10
  COM_WriteSignal13 : Lib_ICAT_VCU_Com/COM_WriteSignal  PARAM_ID=APP_TX_VCU_MCU_HANDBRAKESIGNAL_TX2_3
  COM_WriteSignal14 : Lib_ICAT_VCU_Com/COM_WriteSignal  PARAM_ID=APP_TX_VCU_MCU_FOOTBRAKESIGNAL_TX2_4
  COM_WriteSignal15 : Lib_ICAT_VCU_Com/COM_WriteSignal  PARAM_ID=APP_TX_VCU_MCU_GEARSTATUS_TX2_5
  COM_WriteSignal16 : Lib_ICAT_VCU_Com/COM_WriteSignal  PARAM_ID=APP_TX_VCU_BMS_HV_POWERCMD_TX3_2
  COM_WriteSignal2 : Lib_ICAT_VCU_Com/COM_WriteSignal  PARAM_ID=APP_TX_VCU_MCU_INVERTERCOMMAND_TX1_13
  COM_WriteSignal3 : Lib_ICAT_VCU_Com/COM_WriteSignal  PARAM_ID=APP_TX_VCU_AUX_OILPUMP_COMMAND_TX4_2
  COM_WriteSignal4 : Lib_ICAT_VCU_Com/COM_WriteSignal  PARAM_ID=APP_TX_VCU_AUX_DC_DC_COMMAND_TX4_3
  COM_WriteSignal5 : Lib_ICAT_VCU_Com/COM_WriteSignal  PARAM_ID=APP_TX_VCU_MCU_DRIVENCOMMAND_TX1_12
  COM_WriteSignal6 : Lib_ICAT_VCU_Com/COM_WriteSignal  PARAM_ID=APP_TX_VCU_HMI_VEHICLESTATUS_TX10_1
  COM_WriteSignal7 : Lib_ICAT_VCU_Com/COM_WriteSignal  PARAM_ID=APP_TX_VCU_MCU_ENABLE_TX1_15
  COM_WriteSignal8 : Lib_ICAT_VCU_Com/COM_WriteSignal  PARAM_ID=APP_TX_VCU_MCU_MODECONTROL_TX1_14
  COM_WriteSignal9 : Lib_ICAT_VCU_Com/COM_WriteSignal  PARAM_ID=APP_TX_VCU_MCU_K2CLOSEREQUEST_TX1_4
  Chart : Stateflow chart  TreatAsAtomicUnit=on
  Constant{,3..7} (6 alike) : Constant  Value=0
  Constant1 : Constant  Value=0  OutDataTypeStr=boolean
  Constant2 : Constant
  Constant8 : Constant
  Drivend : Constant
  Gear Status : Constant
  IO_ReadDigitalInput : Lib_ICAT_VCU_IO/IO_ReadDigitalInput  PARAM_ID=ECU_BRAKE_DI_P29
  IO_ReadDigitalInput1 : Lib_ICAT_VCU_IO/IO_ReadDigitalInput  PARAM_ID=ECU_ESTOP_DI_P7
  If : If  NumInputs=5  IfExpression=((u1 == 1) & (u2 == 2) & (u3 == 1) & (u4 == 0) & (u5 == 0))  ElseIfExpressions=((u1 == 2) & (u2 == 2) & (u3 == 1) & (u4 == 0) & (u5 == 0))
  If Action Subsystem : Subsystem  TreatAsAtomicUnit=on
  If Action Subsystem1 : Subsystem  TreatAsAtomicUnit=on
  If Action Subsystem2 : Subsystem  TreatAsAtomicUnit=on
  Invalid : Constant  Value=0
  Merge : Merge  Inputs=3
  Mode Control : Constant  Value=0  OutDataTypeStr=boolean
  OFF : Constant  Value=85  OutDataTypeStr=uint8
  OFF1 : Constant  Value=0  OutDataTypeStr=uint8
  ON : Constant  Value=170  OutDataTypeStr=uint8
  ON1 : Constant  OutDataTypeStr=uint8
  SMFaultMgnt : Subsystem
  Saturation2 : Saturate  UpperLimit=501  LowerLimit=0
  Switch : Switch  Criteria=u2 > Threshold
  Switch1 : Switch  Criteria=u2 > Threshold
  Switch2 : Switch  Criteria=u2 > Threshold
  Terminator1 : Terminator
  Terminator2 : Terminator
  Terminator3 : Terminator
  Motor_RPM : Outport
  wires:
  FaultsINP/1 -> SMFaultMgnt/1(FaultsINP)
  SMFaultMgnt/1(FaultsOut) -> [FaultINP]
  [FaultINP] -> Bus Selector/1
  Bus Selector/1 -> [IdleFault]  "<IdleFault>"
  [IdleFault] -> Chart/11(IdleFault)
  Bus Selector/2 -> [DisRdyFault]  "<DisRdyFault>"
  [DisRdyFault] -> Chart/4(DisRdyFault)
  Bus Selector/3 -> [ChargeRdyFault]  "<ChargeRdyFault>"
  Bus Selector/4 -> [DisActive]  "<DrivingActiveFault>"
  [DisActive] -> Chart/7(DisActiveFault)
  Bus Selector/5 -> [ChargeActiveIN]  "<ChargeActiveFault>"
  [ChargeActiveIN] -> Chart/12(ChargeActiveFault)
  Bus Selector/6 -> [AllPtFaults]  "<AllPtFaults>"
  [AllPtFaults] -> Chart/8(AllFaults)
  [IdleFault] -> Chart/3(AccRdyFault)
  [ChargeRdyFault] -> Chart/5(ChargeRdyFault)
  [KeyPos] -> Chart/2(KeyPos)
  Constant3/1 -> Chart/6(ProxCharge)
  Constant5/1 -> Chart/10(ChargedCmpt)
  [APS] -> Chart/13(APP)
  Chart/6(DriveStatus) -> [DriveStatus]
  Chart/4(FaultActive) -> [FaultActive]
  Chart/3(DriveActive) -> [DriveActive]
  Chart/2(ChargeActive) -> [ChargeActive]
  Chart/1(VehicleState) -> [VehStatus]
  Chart/5(AccActive) -> [AccActive]
  If/1 -> If Action Subsystem/Action
  If/2 -> If Action Subsystem1/Action
  If/3 -> If Action Subsystem2/Action
  ACPIN/1 -> [TrqCmnd]
  [TrqCmnd] -> If Action Subsystem/1(TrqCmnd)
  GearStatus/1 -> [GearStatus]
  [GearStatus] -> If Action Subsystem/2(GearStatus)
  If Action Subsystem/1(TrqToMCU) -> Merge/1
  If Action Subsystem1/1(Out1) -> Merge/2
  If Action Subsystem2/1(Out1) -> Merge/3
  [DriveStatus] -> If/1
  [VehStatus] -> If/2
  [DriveActive] -> If/3
  [ChargeActive] -> If/4
  [FaultActive] -> If/5
  APS/1 -> [APS]
  [MotorRPM] -> Chart/14(MotorRPM)
  KeyPos/1 -> [KeyPos]
  [AccActive] -> Switch/2
  Constant/1 -> IO_ReadDigitalInput/1
  Constant2/1 -> IO_ReadDigitalInput/2
  IO_ReadDigitalInput/2 -> Terminator1/1
  ON/1 -> Switch/1
  OFF/1 -> Switch/3
  Switch/1 -> COM_WriteSignal/1, COM_WriteSignal4/1, COM_WriteSignal3/1
  Chart/7(MCUVehStatus) -> [MCUVehStatus]
  [DriveActive] -> Switch1/2
  Invalid/1 -> Switch1/3
  Drivend/1 -> Switch1/1
  Switch1/1 -> COM_WriteSignal5/1, COM_WriteSignal7/1, COM_WriteSignal11/1, COM_WriteSignal10/1, COM_WriteSignal9/1
  Chart/8(MCUInvCmd) -> [MCUInvCmd]
  Mode Control/1 -> COM_WriteSignal8/1
  Merge/1 -> Saturation2/1
  Constant6/1 -> IO_ReadDigitalInput1/2
  Constant4/1 -> IO_ReadDigitalInput1/1
  IO_ReadDigitalInput1/2 -> Terminator2/1
  IO_ReadDigitalInput1/1 -> COM_WriteSignal12/1
  Constant1/1 -> [HndBrake]
  [HndBrake] -> Chart/1(HndBrake)
  [HndBrake] -> COM_WriteSignal13/1
  IO_ReadDigitalInput/1 -> [FootBrake]
  [FootBrake] -> Chart/9(FootBrake)
  [FootBrake] -> COM_WriteSignal14/1
  Gear Status/1 -> COM_WriteSignal15/1
  Constant7/1 -> COM_ReadSignal/1
  COM_ReadSignal/2 -> Terminator3/1
  Constant8/1 -> COM_ReadSignal/2
  [MotorRPM] -> If Action Subsystem/3(MotorRPM)
  COM_ReadSignal/1 -> Motor_RPM/1, [MotorRPM]
  OFF1/1 -> Switch2/3
  ON1/1 -> Switch2/1
  [AccActive] -> Switch2/2
  Switch2/1 -> COM_WriteSignal16/1
  [MCUVehStatus] -> COM_WriteSignal6/1
  [MCUInvCmd] -> COM_WriteSignal2/1
  Saturation2/1 -> COM_WriteSignal1/1

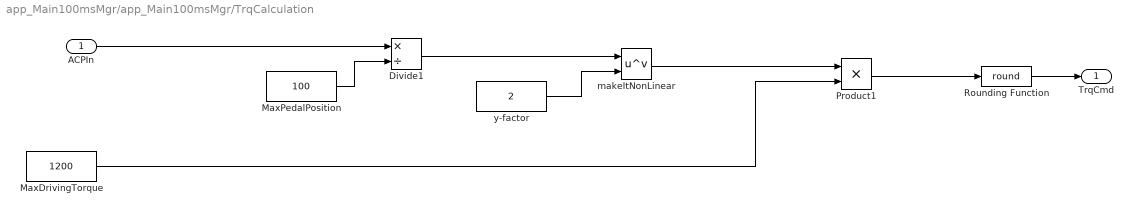
== system app_Main100msMgr/app_Main100msMgr/TrqCalculation ==
  ACPIn : Inport
  Divide1 : Product  Inputs=*/
  MaxDrivingTorque : Constant  Value=1200
  MaxPedalPosition : Constant  Value=100
  Product1 : Product
  Rounding Function : Rounding  Operator=round
  makeItNonLinear : Math  Operator=pow  SaturateOnIntegerOverflow=on
  y-factor : Constant  Value=2
  TrqCmd : Outport
  wires:
  Rounding Function/1 -> TrqCmd/1
  MaxDrivingTorque/1 -> Product1/2
  y-factor/1 -> makeItNonLinear/2
  ACPIn/1 -> Divide1/1
  MaxPedalPosition/1 -> Divide1/2
  makeItNonLinear/1 -> Product1/1
  Product1/1 -> Rounding Function/1
  Divide1/1 -> makeItNonLinear/1

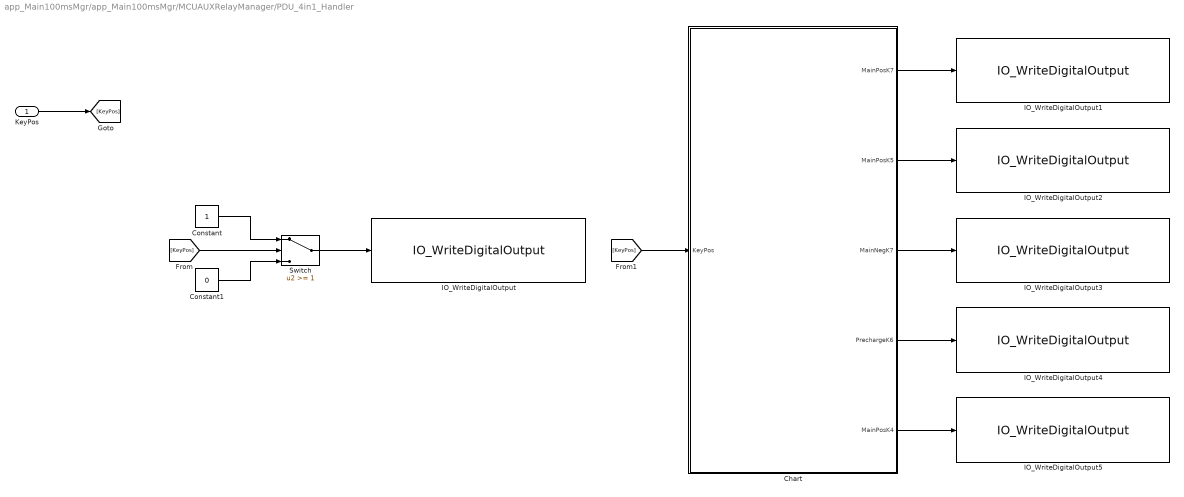
== system app_Main100msMgr/app_Main100msMgr/MCUAUXRelayManager/PDU_4in1_Handler ==
  KeyPos : Inport
  Chart : Stateflow chart  TreatAsAtomicUnit=on
  Constant : Constant
  Constant1 : Constant  Value=0
  IO_WriteDigitalOutput : Lib_ICAT_VCU_IO/IO_WriteDigitalOutput  PARAM_ID=ECU_MCU_Wakeup_ACC_P15
  IO_WriteDigitalOutput1 : Lib_ICAT_VCU_IO/IO_WriteDigitalOutput  PARAM_ID=ECU_K7_POS_Relay_P33
  IO_WriteDigitalOutput2 : Lib_ICAT_VCU_IO/IO_WriteDigitalOutput  PARAM_ID=ECU_K5_Relay_P22
  IO_WriteDigitalOutput3 : Lib_ICAT_VCU_IO/IO_WriteDigitalOutput  PARAM_ID=ECU_K7_NEG_Relay_P34
  IO_WriteDigitalOutput4 : Lib_ICAT_VCU_IO/IO_WriteDigitalOutput  PARAM_ID=ECU_K6_Relay_P24
  IO_WriteDigitalOutput5 : Lib_ICAT_VCU_IO/IO_WriteDigitalOutput  PARAM_ID=ECU_K4_P40
  Switch : Switch  Threshold=1
  wires:
  Switch/1 -> IO_WriteDigitalOutput/1
  [KeyPos] -> Switch/2
  [KeyPos] -> Chart/1(KeyPos)
  Constant1/1 -> Switch/3
  KeyPos/1 -> [KeyPos]
  Chart/2(MainPosK5) -> IO_WriteDigitalOutput2/1
  Chart/3(MainNegK7) -> IO_WriteDigitalOutput3/1
  Constant/1 -> Switch/1
  Chart/1(MainPosK7) -> IO_WriteDigitalOutput1/1
  Chart/4(PrechargeK6) -> IO_WriteDigitalOutput4/1
  Chart/5(MainPosK4) -> IO_WriteDigitalOutput5/1

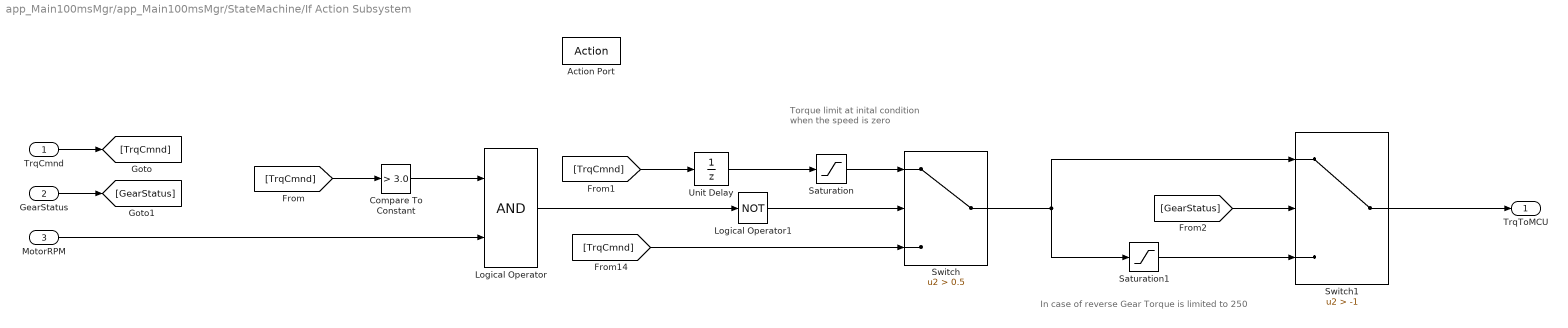
== system app_Main100msMgr/app_Main100msMgr/StateMachine/If Action Subsystem ==
  note: In case of reverse Gear Torque is limited to 250
  note: Torque limit at inital
      | condition when the speed is zero
  TrqCmnd : Inport
  GearStatus : Inport  Port=2
  MotorRPM : Inport  Port=3
  Action Port : ActionPort  ActionType=then
  Compare To Constant : simulink/Logic and Bit Operations/Compare To Constant  relop=>  const=3.0  OutDataTypeStr=boolean
  Logical Operator : Logic  AllPortsSameDT=off  OutDataTypeStr=boolean
  Logical Operator1 : Logic  Operator=NOT  Inputs=1  AllPortsSameDT=off  OutDataTypeStr=boolean
  Saturation : Saturate  UpperLimit=501  LowerLimit=0
  Saturation1 : Saturate  UpperLimit=250  LowerLimit=0
  Switch : Switch  Criteria=u2 > Threshold  Threshold=0.5
  Switch1 : Switch  Criteria=u2 > Threshold  Threshold=-1
  Unit Delay : UnitDelay  InitialCondition=3  SampleTime=-1
  TrqToMCU : Outport
  wires:
  MotorRPM/1 -> Logical Operator/2
  Compare To Constant/1 -> Logical Operator/1
  Logical Operator/1 -> Logical Operator1/1
  TrqCmnd/1 -> [TrqCmnd]
  [TrqCmnd] -> Switch/3
  [TrqCmnd] -> Unit Delay/1
  [TrqCmnd] -> Compare To Constant/1
  Unit Delay/1 -> Saturation/1
  Saturation/1 -> Switch/1
  GearStatus/1 -> [GearStatus]
  [GearStatus] -> Switch1/2
  Switch/1 -> Switch1/1, Saturation1/1
  Saturation1/1 -> Switch1/3
  Switch1/1 -> TrqToMCU/1
  Logical Operator1/1 -> Switch/2

== system app_Main100msMgr/app_Main100msMgr/StateMachine/If Action Subsystem1 ==
  note: Sending zero torque command in case of coasting or braking condition
  Action Port : ActionPort  ActionType=elseif
  ZeroTrq : Constant  Value=0
  Out1 : Outport
  wires:
  ZeroTrq/1 -> Out1/1

== system app_Main100msMgr/app_Main100msMgr/StateMachine/If Action Subsystem2 ==
  note: Sending zero torque command in case of other states
  Action Port : ActionPort  ActionType=else
  Constant : Constant  Value=0
  Out1 : Outport
  wires:
  Constant/1 -> Out1/1
